simulink model "Fig314"  (R2014b)
settings: Solver=ode3  StartTime=0.0  StopTime=5.24288  FixedStep=2e-6  RelTol=1e-5
libraries: commanapbnd3 x1, commrandsrc2 x1
settings Model: Creator=Dennis Silage  LastModifiedBy=Silage
settings DataIOCC: SignalLoggingSaveFormat=ModelDataLogs
settings OptimizationCC: ExpressionDepthLimit=2147483647  InitFltsAndDblsToZero=on
settings DebuggingCC: UnderspecifiedInitializationDetection=Classic  MergeDetectMultiDrivingBlocksExec=none  SolverPrmCheckMsg=none  FcnCallInpInsideContextMsg=UseLocalSettings  StateNameClashWarn=warning
settings GRTTargetCC: CombineOutputUpdateFcns=off  GRTInterface=on

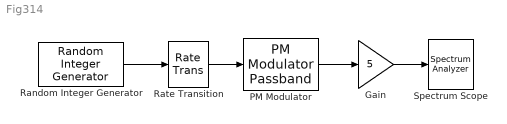
== system Fig314 ==
  Gain : Gain  Gain=5
  PM Modulator : commanapbnd3/PM Modulator Passband  Fc=20000  Ph=pi  Kc=pi
  Random Integer Generator : commrandsrc2/Random Integer Generator  mul=2  seed=randseed  Ts=1e-3  frameBased=off  sampPerFrame=50  orient=on  outDataType=double
  Rate Transition : RateTransition  OutPortSampleTime=2e-6
  Spectrum Scope : SpectrumAnalyzer
  wires:
  Rate Transition/1 -> PM Modulator/1
  Random Integer Generator/1 -> Rate Transition/1
  PM Modulator/1 -> Gain/1
  Gain/1 -> Spectrum Scope/1
